simulink model "L_sys_1var"  (R2019b)
settings: Solver=VariableStepAuto  StartTime=0.0  StopTime=10.0  RelTol=1e-3
undefined symbols (not defined in the file): A_Obs, B_Obs, C_Obs, D_Obs, g, J, K, l, m, Mcart, Noise, Observer
libraries: simulink x1
settings Model: Creator=huojiaxi  LastModifiedBy=huojiaxi
settings DebuggingCC: AlgebraicLoopMsg=none

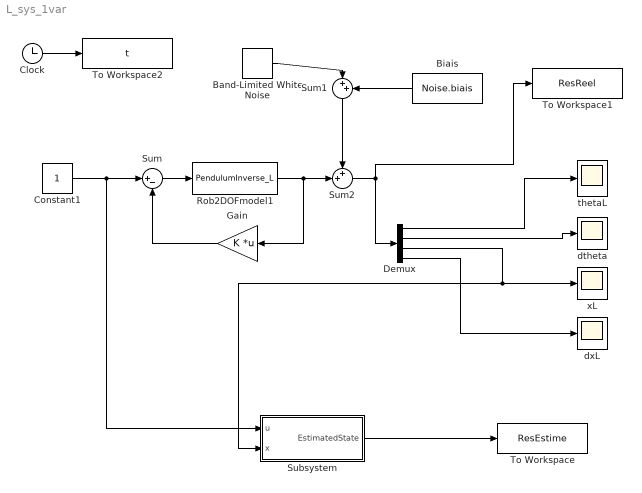
== system L_sys_1var ==
  Band-Limited White Noise : simulink/Sources/Band-Limited White Noise  Cov=Noise.power  Ts=Noise.sampling  seed=Noise.seed
  Biais : Constant  Value=Noise.biais
  Clock : Clock
  Constant1 : Constant
  Demux : Demux
  Gain : Gain  Gain=K  Multiplication=Matrix(K*u) (u vector)
  Rob2DOFmodel1 : S-Function  FunctionName=PendulumInverse_L  Parameters=Mcart,m,l,g,J  SFunctionDeploymentMode=off  EnableBusSupport=off
  Subsystem : Subsystem
  Sum : Sum  Inputs=|+-
  Sum1 : Sum  Inputs=|++
  Sum2 : Sum  Inputs=++|
  To Workspace : ToWorkspace  VariableName=ResEstime  SampleTime=-1
  To Workspace1 : ToWorkspace  VariableName=ResReel  SampleTime=-1
  To Workspace2 : ToWorkspace  VariableName=t  SaveFormat=Timeseries  SampleTime=-1
  dtheta : Scope
  "dxL " : Scope
  thetaL : Scope
  xL : Scope
  wires:
  Clock/1 -> To Workspace2/1
  Demux/4 -> "dxL "/1
  Band-Limited White Noise/1 -> Sum1/1
  Sum2/1 -> Demux/1, To Workspace1/1
  Demux/1 -> thetaL/1
  Rob2DOFmodel1/1 -> Gain/1, Sum2/2
  Demux/3 -> xL/1, Subsystem/2("x ")
  Demux/2 -> dtheta/1
  Sum1/1 -> Sum2/1
  Constant1/1 -> Sum/1, Subsystem/1(u)
  Gain/1 -> Sum/2
  Biais/1 -> Sum1/2
  Sum/1 -> Rob2DOFmodel1/1
  Subsystem/1(EstimatedState) -> To Workspace/1

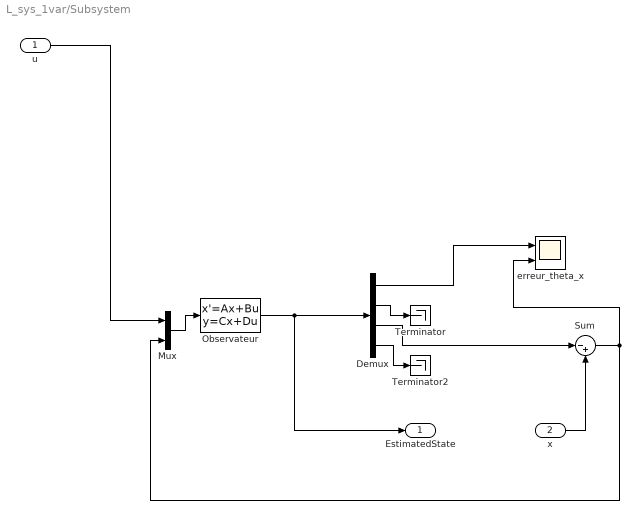
== system L_sys_1var/Subsystem ==
  u : Inport
  "x " : Inport  Port=2
  Demux : Demux
  Mux : Mux  Inputs=2
  Observateur : StateSpace  A=A_Obs  B=B_Obs  C=C_Obs  D=D_Obs  InitialCondition=Observer.IC
  Sum : Sum  Inputs=|-+
  Terminator : Terminator
  Terminator2 : Terminator
  erreur_theta_x : Scope  NumInputPorts=2
  EstimatedState : Outport  VectorParamsAs1DForOutWhenUnconnected=off
  wires:
  Demux/3 -> Sum/1
  Demux/2 -> Terminator/1
  Mux/1 -> Observateur/1
  u/1 -> Mux/1
  Demux/1 -> erreur_theta_x/1
  Observateur/1 -> EstimatedState/1, Demux/1
  Demux/4 -> Terminator2/1
  "x "/1 -> Sum/2
  Sum/1 -> Mux/2, erreur_theta_x/2
